simulink model "flux_tuning"  (R2024a)
settings: Solver=VariableStepAuto  StartTime=0.0  StopTime=0.3  FixedStep=1e-6  MaxStep=1e-3  RelTol=1e-3
values from neighbouring files (symbols this model uses):
  B = 0.068    [parameters.m]
  J = 0.51    [parameters.m]
  Psisn = 1.48    [parameters.m]
  Vac = 230    [parameters.m]
libraries: DEMDlib x6
settings Model: Creator=roberto  LastModifiedBy=roberto
settings DebuggingCC: ReadBeforeWriteMsg=DisableAll  WriteAfterWriteMsg=DisableAll  WriteAfterReadMsg=DisableAll  MultiTaskDSMMsg=none
settings ModelReferenceCC: UpdateModelReferenceTargets=IfOutOfDate
settings SFSimCC: SFSimEcho=off

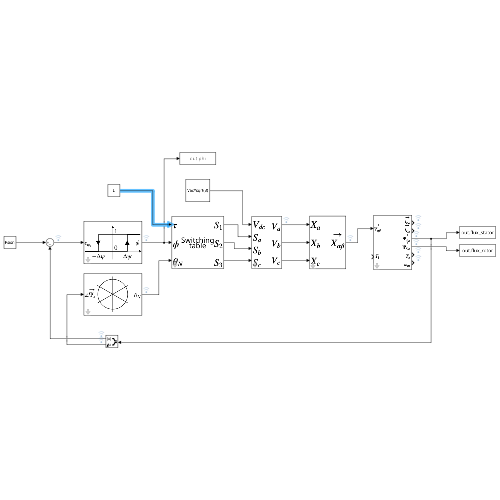
[thumbnail: Simulink's stored preview of the top-level diagram]
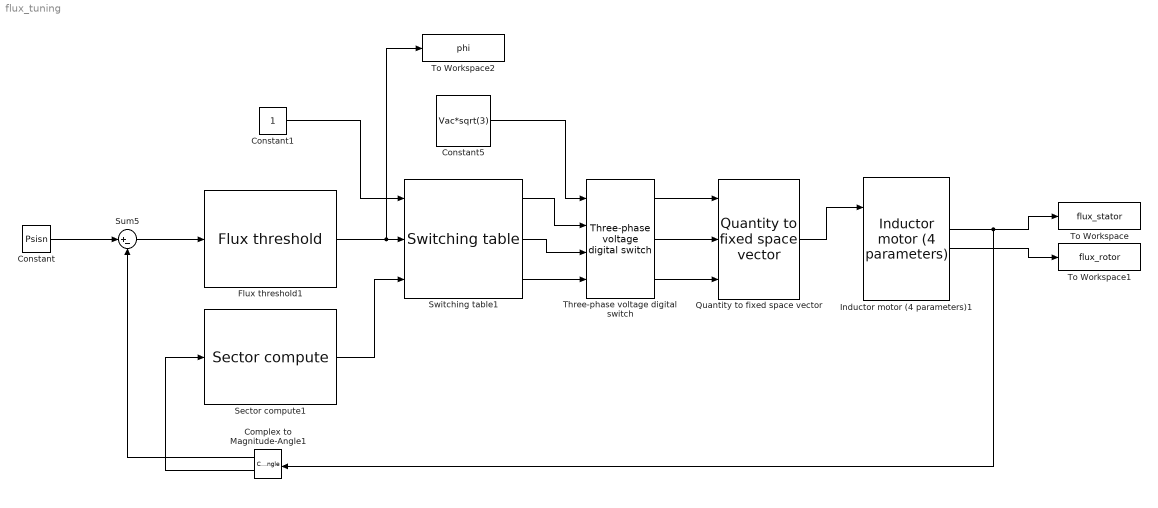
== system flux_tuning ==
  Complex to Magnitude-Angle1 : ComplexToMagnitudeAngle
  Constant : Constant  Value=Psisn
  Constant1 : Constant
  Constant5 : Constant  Value=Vac*sqrt(3)
  Flux threshold1 : DEMDlib/DTC/Flux threshold  dpsi=dPsi
      settings: SourceProductName=DEMD
  Inductor motor (4 parameters)1 : DEMDlib/Inductor motor (4 parameters)  Rs=Rs  Lks=Lks  Rr=Rkr  Lm=Lkm  np=np  J=J  B=B
      settings: SourceProductName=DEMD
  Quantity to fixed space vector : DEMDlib/Quantity to fixed space vector
      settings: SourceProductName=DEMD
  Sector compute1 : DEMDlib/DTC/Sector compute
      settings: SourceProductName=DEMD
  Sum5 : Sum  Inputs=|+-
  Switching table1 : DEMDlib/DTC/Switching table
      settings: SourceProductName=DEMD
  Three-phase voltage digital switch : DEMDlib/Three-phase voltage digital switch
      settings: SourceProductName=DEMD
  To Workspace : ToWorkspace  VariableName=flux_stator  SaveFormat=Timeseries  SampleTime=-1
  To Workspace1 : ToWorkspace  VariableName=flux_rotor  SaveFormat=Timeseries  SampleTime=-1
  To Workspace2 : ToWorkspace  VariableName=phi  SaveFormat=Timeseries  SampleTime=-1
  wires:
  Quantity to fixed space vector/1 -> Inductor motor (4 parameters)1/1
  Sector compute1/1 -> Switching table1/3
  Flux threshold1/1 -> To Workspace2/1, Switching table1/2
  Sum5/1 -> Flux threshold1/1
  Constant/1 -> Sum5/1
  Inductor motor (4 parameters)1/3 -> Complex to Magnitude-Angle1/1, To Workspace/1
  Complex to Magnitude-Angle1/1 -> Sum5/2
  Complex to Magnitude-Angle1/2 -> Sector compute1/1
  Switching table1/3 -> Three-phase voltage digital switch/4
  Switching table1/2 -> Three-phase voltage digital switch/3
  Switching table1/1 -> Three-phase voltage digital switch/2
  Constant5/1 -> Three-phase voltage digital switch/1
  Three-phase voltage digital switch/1 -> Quantity to fixed space vector/1
  Three-phase voltage digital switch/2 -> Quantity to fixed space vector/2
  Three-phase voltage digital switch/3 -> Quantity to fixed space vector/3
  Inductor motor (4 parameters)1/4 -> To Workspace1/1
  Constant1/1 -> Switching table1/1
